simulink model "zadacha_17"  (Simulink 7.1)
settings: Solver=ode45  StartTime=0.0  StopTime=20  RelTol=1e-3
settings Model: Creator=Slavi  LastModifiedBy=Slavi

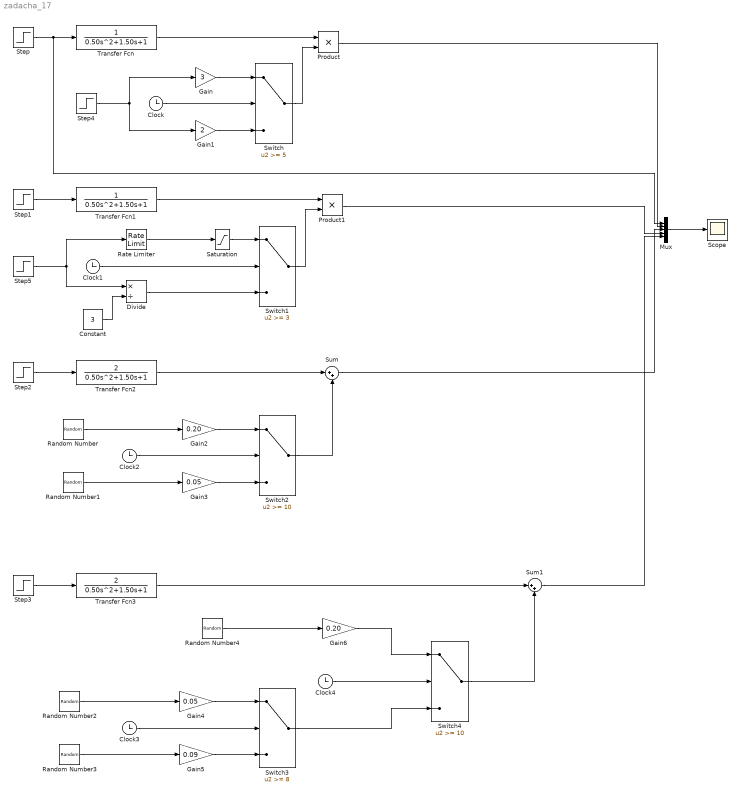
== system zadacha_17 ==
  Clock{,1..4} (5 alike) : Clock
      settings: Decimation=10
  Constant : Constant  Value=3  OutDataType=sfix(16)  OutScaling=2^0
  Divide : Product  Inputs=*/  OutDataType=sfix(16)  OutScaling=2^-10  SaturateOnIntegerOverflow=on  InputSameDT=on
  Gain : Gain  Gain=3  ParameterDataType=sfix(16)  ParameterScaling=2^0  OutDataType=sfix(16)  OutScaling=2^0
  Gain1 : Gain  Gain=2  ParameterDataType=sfix(16)  ParameterScaling=2^0  OutDataType=sfix(16)  OutScaling=2^0
  Gain2 : Gain  Gain=0.20  ParameterDataType=sfix(16)  ParameterScaling=2^0  OutDataType=sfix(16)  OutScaling=2^0
  Gain3 : Gain  Gain=0.05  ParameterDataType=sfix(16)  ParameterScaling=2^0  OutDataType=sfix(16)  OutScaling=2^0
  Gain4 : Gain  Gain=0.05  ParameterDataType=sfix(16)  ParameterScaling=2^0  OutDataType=sfix(16)  OutScaling=2^0
  Gain5 : Gain  Gain=0.09  ParameterDataType=sfix(16)  ParameterScaling=2^0  OutDataType=sfix(16)  OutScaling=2^0
  Gain6 : Gain  Gain=0.20  ParameterDataType=sfix(16)  ParameterScaling=2^0  OutDataType=sfix(16)  OutScaling=2^0
  Mux : Mux  Inputs=5
  Product : Product  OutDataType=sfix(16)  OutScaling=2^0  RndMeth=Zero
  Product1 : Product  OutDataType=sfix(16)  OutScaling=2^0  RndMeth=Zero
  Random Number{,1..4} (5 alike) : RandomNumber  SampleTime=0
  Rate Limiter : RateLimiter
  Saturation : Saturate  UpperLimit=6  LowerLimit=2  OutDataType=sfix(16)  OutScaling=2^0
  Scope : Scope
  Step{,1..2,4} (4 alike) : Step  Time=0
  Step3 : Step  SampleTime=0
  Step5 : Step  Time=0  After=6
  Sum : Sum  Inputs=|++  OutDataType=sfix(16)  OutScaling=2^0
  Sum1 : Sum  Inputs=|++  OutDataType=sfix(16)  OutScaling=2^0
  Switch : Switch  Threshold=5  OutDataType=sfix(16)  OutScaling=2^0  SaturateOnIntegerOverflow=on  InputSameDT=on
  Switch1 : Switch  Threshold=3  OutDataType=sfix(16)  OutScaling=2^0  SaturateOnIntegerOverflow=on  InputSameDT=on
  Switch2 : Switch  Threshold=10  OutDataType=sfix(16)  OutScaling=2^0  SaturateOnIntegerOverflow=on  InputSameDT=on
  Switch3 : Switch  Threshold=8  OutDataType=sfix(16)  OutScaling=2^0  SaturateOnIntegerOverflow=on  InputSameDT=on
  Switch4 : Switch  Threshold=10  OutDataType=sfix(16)  OutScaling=2^0  SaturateOnIntegerOverflow=on  InputSameDT=on
  Transfer Fcn : TransferFcn  Denominator=[0.50 1.50 1]
  Transfer Fcn1 : TransferFcn  Denominator=[0.50 1.50 1]
  Transfer Fcn2 : TransferFcn  Numerator=[2]  Denominator=[0.50 1.50 1]
  Transfer Fcn3 : TransferFcn  Numerator=[2]  Denominator=[0.50 1.50 1]
  wires:
  Step/1 -> Transfer Fcn/1, Mux/1
  Step1/1 -> Transfer Fcn1/1
  Step2/1 -> Transfer Fcn2/1
  Step3/1 -> Transfer Fcn3/1
  Mux/1 -> Scope/1
  Gain/1 -> Switch/1
  Transfer Fcn/1 -> Product/1
  Gain1/1 -> Switch/3
  Clock/1 -> Switch/2
  Switch/1 -> Product/2
  Step4/1 -> Gain/1, Gain1/1
  Divide/1 -> Switch1/3
  Clock1/1 -> Switch1/2
  Switch1/1 -> Product1/2
  Step5/1 -> Rate Limiter/1, Divide/1
  Transfer Fcn1/1 -> Product1/1
  Saturation/1 -> Switch1/1
  Rate Limiter/1 -> Saturation/1
  Constant/1 -> Divide/2
  Product/1 -> Mux/2
  Transfer Fcn2/1 -> Sum/1
  Switch2/1 -> Sum/2
  Clock2/1 -> Switch2/2
  Gain2/1 -> Switch2/1
  Random Number/1 -> Gain2/1
  Random Number1/1 -> Gain3/1
  Gain3/1 -> Switch2/3
  Product1/1 -> Mux/3
  Sum/1 -> Mux/4
  Clock3/1 -> Switch3/2
  Switch3/1 -> Switch4/3
  Clock4/1 -> Switch4/2
  Random Number2/1 -> Gain4/1
  Random Number3/1 -> Gain5/1
  Gain4/1 -> Switch3/1
  Gain5/1 -> Switch3/3
  Switch4/1 -> Sum1/2
  Transfer Fcn3/1 -> Sum1/1
  Random Number4/1 -> Gain6/1
  Gain6/1 -> Switch4/1
  Sum1/1 -> Mux/5
